simulink model "s2"  (Simulink 2.00)
settings: Solver=ode15s  StartTime=0.0  StopTime=5  MaxStep=0.005  RelTol=1e-6  AbsTol=1e-6
values from neighbouring files (symbols this model uses):
  D = 0.0    (= 0)    [M2.M]    (also in M3A.M; M3B.M)
  J = 0.8    [M1.M]    (also in M2.M = 2.5; M3A.M = 0.5; M3B.M = 0.5; M4.M = 0.015)
  Laq = 0.018    [M1.M]    (also in M2.M = 0.012; M3A.M; M3B.M; M4.M = 0.01)
  Ra = 0.24    [M1.M]    (also in M2.M = 0.3; M3A.M = 0.14; M3B.M = 0.14; M4.M = 0.6)
settings Model: SaveTime=off  SaveOutput=off  ConsistencyChecking=off

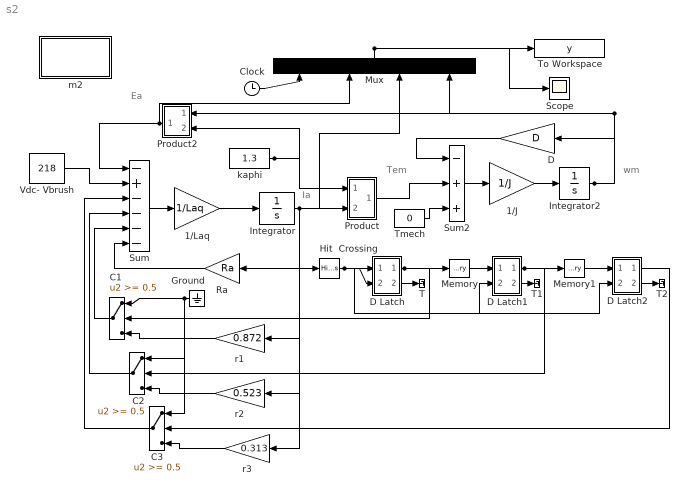
== system s2 ==
  note: Ia
  note: Tem
  note: Ea
  note: wm
  1/J : Gain  Gain=1/J
  1/Laq : Gain  Gain=1/Laq
  C1 : Switch  Orientation=left  Threshold=0.5
  C2 : Switch  Orientation=left  Threshold=0.5
  C3 : Switch  Orientation=left  Threshold=0.5
  Clock : Clock
      settings: DeleteFcn=simclock BlockIsBeingDestroyed  PostSaveFcn=simclock Save
  D : Gain  Orientation=left  Gain=D
  D Latch : Subsystem
  D Latch1 : Subsystem
  D Latch2 : Subsystem
  Ground : Ground  Orientation=left
  Hit  Crossing : HitCross  HitCrossingOffset=60  HitCrossingDirection=falling  ShowOutputPort=on
  Integrator : Integrator  ExternalReset=none  InitialConditionSource=internal  InitialCondition=0  LimitOutput=off  UpperSaturationLimit=inf  LowerSaturationLimit=-inf  ShowSaturationPort=off  ShowStatePort=off  AbsoluteTolerance=auto
  Integrator2 : Integrator  ExternalReset=none  InitialConditionSource=internal  InitialCondition=0  LimitOutput=off  UpperSaturationLimit=inf  LowerSaturationLimit=-inf  ShowSaturationPort=off  ShowStatePort=off  AbsoluteTolerance=auto
  m2 : Subsystem
      settings: OpenFcn=m2
      mask Type: Masked block of m2.m
      mask Help: Uses m2.m to initialize and plot
      mask Display: disp('Initialize\nand plot')
  Memory : Memory  X0=0  InheritSampleTime=off
  Memory1 : Memory  X0=0  InheritSampleTime=off
  Mux : Mux  Orientation=up  Inputs=4
  Product : Subsystem
      mask Type: Dot Product
      mask Description:
      | Inner (dot) product.
      | y=sum(u1.*u2)
      mask Help: Computes the inner (dot) product of the inputs: sum(u1.*u2).  The inputs are vectors of the same length. Output is a scalar.
      mask Display: disp('.\n')
  Product2 : Subsystem  Orientation=left
      mask Type: Dot Product
      mask Description:
      | Inner (dot) product.
      | y=sum(u1.*u2)
      mask Help: Computes the inner (dot) product of the inputs: sum(u1.*u2).  The inputs are vectors of the same length. Output is a scalar.
      mask Display: disp('.\n')
  Ra : Gain  Orientation=left  Gain=Ra
  Scope : Scope
      settings: TickLabels=on  TimeRange=auto  YMin=-10  YMax=250  SaveToWorkspace=off  SaveName=ScopeData  LimitMaxRows=off
  Sum : Sum  Inputs=-+----
  Sum2 : Sum  Inputs=-++
  T : Terminator
  T1 : Terminator
  T2 : Terminator
  Tmech : Constant  Value=0
  To Workspace : ToWorkspace  VariableName=y  SampleTime=0
      settings: Buffer=2000
  Vdc- Vbrush : Constant  Value=218
  kaphi : Constant  Value=1.3
  r1 : Gain  Orientation=left  Gain=0.872
  r2 : Gain  Orientation=left  Gain=0.523
  r3 : Gain  Orientation=left  Gain=0.313
  wires:
  Integrator2/1 -> Mux/4, D/1, Product2/1(in_1)
  r3/1 -> C3/3
  r2/1 -> C2/3
  r1/1 -> C1/3
  C1/1 -> Sum/5
  C2/1 -> Sum/4
  C3/1 -> Sum/3
  Clock/1 -> Mux/1
  Mux/1 -> Scope/1, To Workspace/1
  Tmech/1 -> Sum2/3
  Product/1(out_1) -> Sum2/2
  Ra/1 -> Sum/6
  Integrator/1 -> r3/1, r2/1, r1/1, Hit  Crossing/1, Ra/1, Mux/3, Product/2(in_2)
  Vdc- Vbrush/1 -> Sum/2
  1/Laq/1 -> Integrator/1
  D/1 -> Sum2/1
  kaphi/1 -> Product/1(in_1), Product2/2(in_2)
  1/J/1 -> Integrator2/1
  Sum2/1 -> 1/J/1
  Sum/1 -> 1/Laq/1
  Memory/1 -> D Latch1/1(D)
  Memory1/1 -> D Latch2/1(D)
  Hit  Crossing/1 -> D Latch/1(D), D Latch/2(C), D Latch1/2(C), D Latch2/2(C)
  D Latch2/1(Q) -> C3/2
  D Latch1/1(Q) -> Memory1/1, C2/2
  D Latch/1(Q) -> Memory/1, C1/2
  Product2/1(out_1) -> Sum/1, Mux/2
  Ground/1 -> C1/1, C2/1, C3/1
  D Latch/2(!Q) -> T/1
  D Latch1/2(!Q) -> T1/1
  D Latch2/2(!Q) -> T2/1

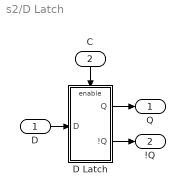
== system s2/D Latch ==
  D : Inport  Port=1  PortWidth=-1  SampleTime=-1
  C : Inport  Orientation=down  Port=2  PortWidth=-1  SampleTime=-1
  D Latch : Subsystem
  Q : Outport  Port=1  InitialOutput=0
  !Q : Outport  Port=2  InitialOutput=1
  wires:
  D Latch/2(!Q) -> !Q/1
  D/1 -> D Latch/1(D)
  D Latch/1(Q) -> Q/1
  C/1 -> D Latch/Enable

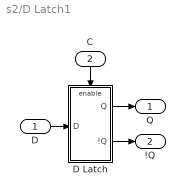
== system s2/D Latch1 ==
  D : Inport  Port=1  PortWidth=-1  SampleTime=-1
  C : Inport  Orientation=down  Port=2  PortWidth=-1  SampleTime=-1
  D Latch : Subsystem
  Q : Outport  Port=1  InitialOutput=0
  !Q : Outport  Port=2  InitialOutput=1
  wires:
  D Latch/2(!Q) -> !Q/1
  D/1 -> D Latch/1(D)
  D Latch/1(Q) -> Q/1
  C/1 -> D Latch/Enable

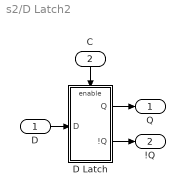
== system s2/D Latch2 ==
  D : Inport  Port=1  PortWidth=-1  SampleTime=-1
  C : Inport  Orientation=down  Port=2  PortWidth=-1  SampleTime=-1
  D Latch : Subsystem
  Q : Outport  Port=1  InitialOutput=0
  !Q : Outport  Port=2  InitialOutput=1
  wires:
  D Latch/2(!Q) -> !Q/1
  D/1 -> D Latch/1(D)
  D Latch/1(Q) -> Q/1
  C/1 -> D Latch/Enable

== system s2/m2 ==
  note: Masked block of m2.m in Chapter 8
      | to initialize s2.m and plot results

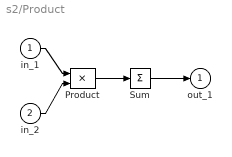
== system s2/Product ==
  in_1 : Inport  Port=1  PortWidth=-1  SampleTime=-1
  in_2 : Inport  Port=2  PortWidth=-1  SampleTime=-1
  Product : Product  Inputs=2
  Sum : Sum  Inputs=+
  out_1 : Outport  Port=1  InitialOutput=0
  wires:
  Sum/1 -> out_1/1
  Product/1 -> Sum/1
  in_1/1 -> Product/1
  in_2/1 -> Product/2

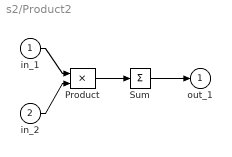
== system s2/Product2 ==
  in_1 : Inport  Port=1  PortWidth=-1  SampleTime=-1
  in_2 : Inport  Port=2  PortWidth=-1  SampleTime=-1
  Product : Product  Inputs=2
  Sum : Sum  Inputs=+
  out_1 : Outport  Port=1  InitialOutput=0
  wires:
  Sum/1 -> out_1/1
  Product/1 -> Sum/1
  in_1/1 -> Product/1
  in_2/1 -> Product/2

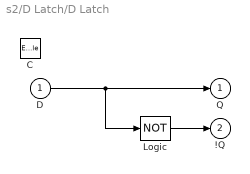
== system s2/D Latch/D Latch ==
  D : Inport  Port=1  PortWidth=-1  SampleTime=-1
  C : EnablePort
  Logic : Logic  Operator=NOT  Inputs=1
  Q : Outport  Port=1  InitialOutput=0
  !Q : Outport  Port=2  InitialOutput=1
  wires:
  D/1 -> Logic/1, Q/1
  Logic/1 -> !Q/1

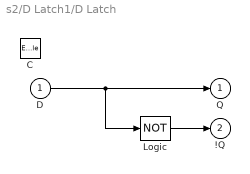
== system s2/D Latch1/D Latch ==
  D : Inport  Port=1  PortWidth=-1  SampleTime=-1
  C : EnablePort
  Logic : Logic  Operator=NOT  Inputs=1
  Q : Outport  Port=1  InitialOutput=0
  !Q : Outport  Port=2  InitialOutput=1
  wires:
  D/1 -> Logic/1, Q/1
  Logic/1 -> !Q/1

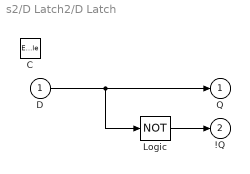
== system s2/D Latch2/D Latch ==
  D : Inport  Port=1  PortWidth=-1  SampleTime=-1
  C : EnablePort
  Logic : Logic  Operator=NOT  Inputs=1
  Q : Outport  Port=1  InitialOutput=0
  !Q : Outport  Port=2  InitialOutput=1
  wires:
  D/1 -> Logic/1, Q/1
  Logic/1 -> !Q/1
